simulink model "sldemo_bus_counter"  (R2020a)
settings: Solver=ode5  StartTime=0.0  StopTime=30  FixedStep=0.1  RelTol=1e-3  EnableMultiTasking=on
InitFcn:
  | warning('off','Simulink:Logging:DatasetRTWGenRootOutputNotSupported');
  | warning('off','Simulink:Logging:DatasetRTWGenStateNotSupported');
StartFcn:
  | warning('off','Simulink:Logging:DatasetRTWGenRootOutputNotSupported');
  | warning('off','Simulink:Logging:DatasetRTWGenStateNotSupported');
StopFcn:
  | warning('on','Simulink:Logging:DatasetRTWGenRootOutputNotSupported');
  | warning('on','Simulink:Logging:DatasetRTWGenStateNotSupported');
PauseFcn:
  | warning('on','Simulink:Logging:DatasetRTWGenRootOutputNotSupported');
  | warning('on','Simulink:Logging:DatasetRTWGenStateNotSupported');
settings Model: ModifiedByFormat=The MathWorks Inc.  ExtModeAutoUpdateStatusClock=off  Creator=The MathWorks, Inc.  LastModifiedBy=The MathWorks Inc.
settings DataIOCC: LimitDataPoints=on  SaveFinalState=on  SaveOutput=off  SaveState=on  SaveTime=off  ReturnWorkspaceOutputs=off  SignalLoggingName=logsOut
settings OptimizationCC: DefaultParameterBehavior=Inlined  InlineInvariantSignals=on  ExpressionDepthLimit=2147483647  InitFltsAndDblsToZero=on  LifeSpan=inf
settings DebuggingCC: SaveWithParameterizedLinksMsg=none  CheckExecutionContextPreStartOutputMsg=on  CheckExecutionContextRuntimeOutputMsg=on  MultiTaskDSMMsg=warning  MultiTaskCondExecSysMsg=none  SigSpecEnsureSampleTimeMsg=none  FcnCallInpInsideContextMsg=warning  RootOutportRequireBusObject=none  AllowSymbolicDim=off  StateNameClashWarn=warning  StrictBusMsg=ErrorOnBusTreatedAsVector  SFUnexpectedBacktrackingDiag=warning  SFNoUnconditionalDefaultTransitionDiag=warning  SFExecutionAtInitializationDiag=none  ArithmeticOperatorsInVariantConditions=warning
settings HardwareCC: ProdBitPerPointer=32  ProdBitPerSizeT=32  ProdBitPerPtrDiffT=32  ProdLargestAtomicFloat=None  ProdIntDivRoundTo=Undefined  ProdEndianess=Unspecified  ProdWordSize=32  ProdHWDeviceType=32-bit Generic  TargetHWDeviceType=32-bit Generic
settings ModelReferenceCC: UpdateModelReferenceTargets=IfOutOfDate  PropagateSignalLabelsOutOfModel=off
settings SFSimCC: SimUseLocalCustomCode=off  CustomCodeUndefinedFunction=UseInterfaceOnly
settings RTWCC: Description=Generic Real-Time Target  RTWUseLocalCustomCode=off
settings CodeAppCC: MaxIdLength=100  StateflowObjectComments=on
settings GRTTargetCC: TargetFcnLib=ansi_tfl_tmw.mat  TargetLangStandard=C89/C90 (ANSI)  CombineOutputUpdateFcns=off  GRTInterface=on
settings ConfigComp: CovMetricSettings=dw  CovHtmlReporting=on  CovSaveCumulativeToWorkspaceVar=on  CovSaveSingleToWorkspaceVar=on  CovExternalEMLEnable=off  CovSFcnEnable=off

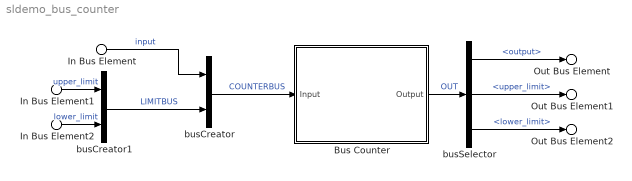
== system sldemo_bus_counter ==
  In Bus Element : Inport  PortName=Input  Element=input
  In Bus Element1 : Inport  PortName=Input  Element=LIMITBUS.upper_limit
  In Bus Element2 : Inport  PortName=Input  Element=LIMITBUS.lower_limit
  Bus Counter : Subsystem  TreatAsAtomicUnit=on
  busCreator : BusCreator  Inputs=2
  busCreator1 : BusCreator  Inputs=2
  busSelector : BusSelector  OutputSignals=output,LIMITBUS.upper_limit,LIMITBUS.lower_limit
  Out Bus Element : Outport  PortName=Output  Element=output
  Out Bus Element1 : Outport  PortName=Output  Element=LIMITBUS.upper_limit
  Out Bus Element2 : Outport  PortName=Output  Element=LIMITBUS.lower_limit
  wires:
  busSelector/3 -> Out Bus Element2/1  "<lower_limit>"
  In Bus Element/1 -> busCreator/1  "input"
  Bus Counter/1(Output) -> busSelector/1  "OUT"
  busSelector/2 -> Out Bus Element1/1  "<upper_limit>"
  busCreator1/1 -> busCreator/2  "LIMITBUS"
  In Bus Element1/1 -> busCreator1/1  "upper_limit"
  busSelector/1 -> Out Bus Element/1  "<output>"
  busCreator/1 -> Bus Counter/1(Input)  "COUNTERBUS"
  In Bus Element2/1 -> busCreator1/2  "lower_limit"

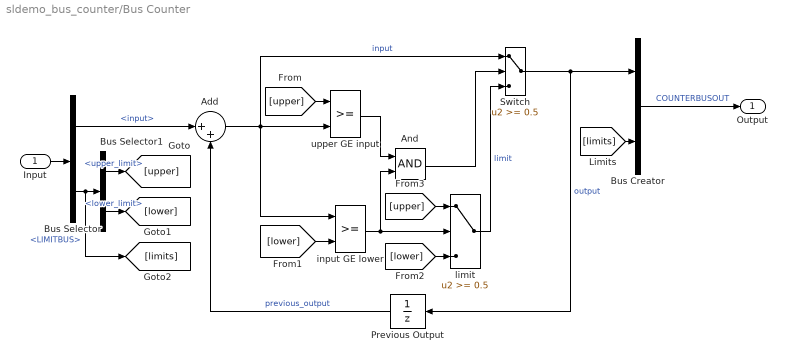
== system sldemo_bus_counter/Bus Counter ==
  Input : Inport
  " input GE lower" : RelationalOperator  Priority=1  OutDataTypeStr=boolean  RndMeth=Nearest  InputSameDT=on
      settings: AttributesFormatString=\n
  " limit" : Switch  Threshold=0.5  SaturateOnIntegerOverflow=on  InputSameDT=on
  Add : Sum  Inputs=|++
  And : Logic  OutDataTypeStr=boolean
  Bus Creator : BusCreator  Inputs=2
  Bus Selector : BusSelector  OutputSignals=input,LIMITBUS
  Bus Selector1 : BusSelector  OutputSignals=upper_limit,lower_limit
  Previous Output : UnitDelay  SampleTime=-1  HasFrameUpgradeWarning=on
  Switch : Switch  Threshold=0.5  SaturateOnIntegerOverflow=on  InputSameDT=on
  upper GE input : RelationalOperator  Priority=0  OutDataTypeStr=boolean  RndMeth=Nearest  InputSameDT=on
      settings: AttributesFormatString=\n
  Output : Outport  VectorParamsAs1DForOutWhenUnconnected=off
  wires:
  [limits] -> Bus Creator/2
  Bus Creator/1 -> Output/1  "COUNTERBUSOUT"
  Bus Selector1/2 -> [lower]  "<lower_limit>"
  Bus Selector1/1 -> [upper]  "<upper_limit>"
  Bus Selector/1 -> Add/1  "<input>"
  Bus Selector/2 -> Bus Selector1/1, [limits]  "<LIMITBUS>"
  Input/1 -> Bus Selector/1
  Add/1 -> " input GE lower"/1, upper GE input/2, Switch/1  "input"
  And/1 -> Switch/2
  " input GE lower"/1 -> And/2, " limit"/2
  [lower] -> " input GE lower"/2
  [upper] -> upper GE input/1
  [lower] -> " limit"/3
  Previous Output/1 -> Add/2  "previous_output"
  upper GE input/1 -> And/1
  " limit"/1 -> Switch/3  "limit"
  Switch/1 -> Bus Creator/1, Previous Output/1  "output"
  [upper] -> " limit"/1
